simulink model "StateOnOffChk"  (R2018b)
settings: Solver=FixedStepDiscrete  StartTime=0.0  StopTime=10.0  FixedStep=0.01  RelTol=1e-3
settings Model: Creator=sn2xws  LastModifiedBy=sn2xws
settings DataIOCC: SaveFormat=StructureWithTime
settings OptimizationCC: DefaultParameterBehavior=Inlined  EnhancedBackFolding=on  PassReuseOutputArgsAs=Individual arguments  ZeroExternalMemoryAtStartup=off  ZeroInternalMemoryAtStartup=off  OptimizeBlockOrder=speed  DifferentSizesBufferReuse=on  OptimizationCustomize=off
settings DebuggingCC: ParameterTunabilityLossMsg=error
settings ModelReferenceCC: ModelReferenceNumInstancesAllowed=Single
settings SFSimCC: MATLABDynamicMemAlloc=off
settings RTWCC: SystemTargetFile=autosar.tlc  GenCodeOnly=on  TemplateMakefile=ert_default_tmf  Description=AUTOSAR  GenerateReport=on  IncludeHyperlinkInReport=on  LaunchReport=on  GenerateTraceInfo=on  GenerateTraceReport=on  GenerateTraceReportSl=on  GenerateTraceReportSf=on  GenerateTraceReportEml=on  GenerateCodeMetricsReport=on
settings CodeAppCC: ForceParamTrailComments=on  IgnoreCustomStorageClasses=off  OperatorAnnotations=on  SimulinkDataObjDesc=on  SFDataObjDesc=on  InsertBlockDesc=on
settings STFCustomTargetCC: TargetLangStandard=C99 (ISO)  MultiwordLength=256  ParMdlRefBuildCompliant=on  CompOptLevelCompliant=on  IncludeMdlTerminateFcn=off  CombineOutputUpdateFcns=on  SuppressErrorStatus=on  ERTCustomFileBanners=on  SupportNonFinite=off  SupportComplex=off  SupportContinuousTime=off  SupportNonInlinedSFcns=off  RemoveResetFunc=on  MATLABClassNameForMDSCustomization=Simulink.SoftwareTarget.ERTCustomization  AutosarCompliant=on  UseToolchainInfoCompliant=on  LookupTableObjectStructAxisOrder=2,1,3,4,...  LUTObjectStructOrderEvenSpacing=Size,Table,Breakpoints  SystemTargetFile=autosar.tlc
settings ERTTargetCC: TargetLangStandard=C99 (ISO)  ConcurrentExecutionCompliant=off  IncludeMdlTerminateFcn=off  SuppressErrorStatus=on  SupportNonFinite=off  SupportComplex=off  ModelStepFunctionPrototypeControlCompliant=off  CPPClassGenCompliant=off  AutosarCompliant=on  LookupTableObjectStructAxisOrder=2,1,3,4,...  LUTObjectStructOrderEvenSpacing=Size,Table,Breakpoints  InlinedParameterPlacement=NonHierarchical  ERTCustomFileTemplate=example_file_process.tlc  ERTFilePackagingFormat=Compact

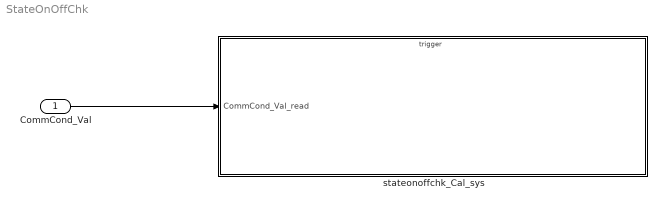
== system StateOnOffChk ==
  CommCond_Val : Inport  OutDataTypeStr=boolean  PortDimensions=1
  stateonoffchk_Cal_sys : Subsystem
  wires:
  CommCond_Val/1 -> stateonoffchk_Cal_sys/1(CommCond_Val_read)

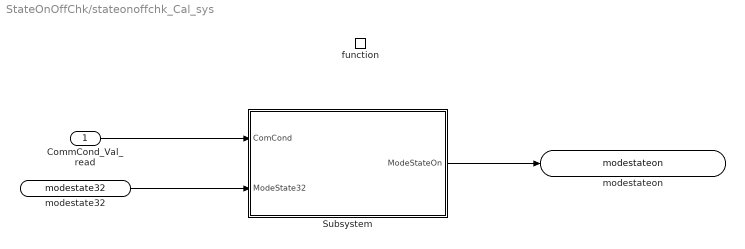
== system StateOnOffChk/stateonoffchk_Cal_sys ==
  CommCond_Val_read : Inport
  function : TriggerPort  TriggerType=function-call  IsSimulinkFunction=on  FunctionName=stateonoffchk_Cal  VariantControl=(inherit)
  Subsystem : Subsystem
  modestate32 : ArgIn  OutDataTypeStr=uint32  ArgumentName=modestate32
  modestateon : ArgOut  OutDataTypeStr=boolean  ArgumentName=modestateon
  wires:
  CommCond_Val_read/1 -> Subsystem/1(ComCond)
  Subsystem/1(ModeStateOn) -> modestateon/1
  modestate32/1 -> Subsystem/2(ModeState32)

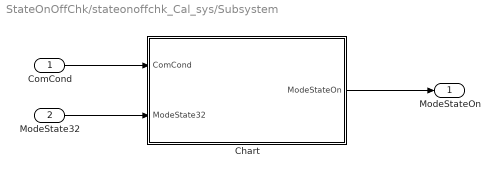
== system StateOnOffChk/stateonoffchk_Cal_sys/Subsystem ==
  ComCond : Inport
  ModeState32 : Inport  Port=2
  Chart : Stateflow chart  TreatAsAtomicUnit=on
  ModeStateOn : Outport
  wires:
  ModeState32/1 -> Chart/2(ModeState32)
  ComCond/1 -> Chart/1(ComCond)
  Chart/1(ModeStateOn) -> ModeStateOn/1

== stateflow chart StateOnOffChk/stateonoffchk_Cal_sys/Subsystem/Chart ==
  state MdStateOff
    en:ModeStateOn=0;
  state MdStateOn
    en:ModeStateOn=1;
  (default) -> MdStateOff
  MdStateOff -> MdStateOn : [ComCond]
  MdStateOn -> MdStateOff : [!ComCond&&ModeState32==0]
  data: ComCond input; ModeState32 input; ModeStateOn output boolean
